simulink model "svpwm"  (R2022b)
settings: Solver=VariableStepAuto  StartTime=0.0  StopTime=10.0  RelTol=1e-3
settings Model: Creator=15403  LastModifiedBy=15403

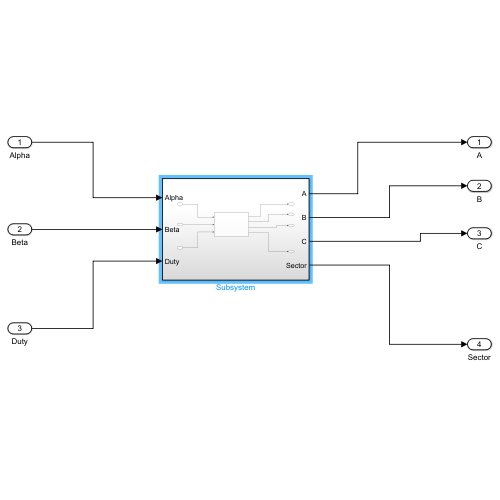
[thumbnail: Simulink's stored preview of the top-level diagram]
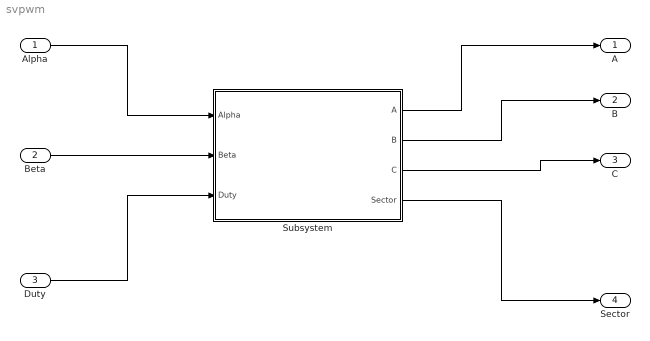
== system svpwm ==
  Alpha : Inport
  Beta : Inport  Port=2
  Duty : Inport  Port=3
  Subsystem : Subsystem
  A : Outport
  B : Outport  Port=2
  C : Outport  Port=3
  Sector : Outport  Port=4
  wires:
  Alpha/1 -> Subsystem/1(Alpha)
  Beta/1 -> Subsystem/2(Beta)
  Duty/1 -> Subsystem/3(Duty)
  Subsystem/1(A) -> A/1
  Subsystem/2(B) -> B/1
  Subsystem/3(C) -> C/1
  Subsystem/4(Sector) -> Sector/1

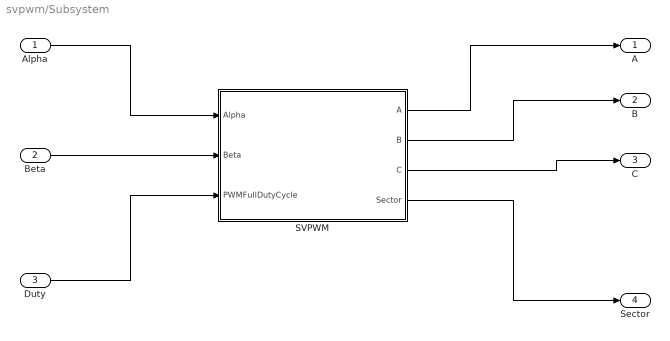
== system svpwm/Subsystem ==
  Alpha : Inport
  Beta : Inport  Port=2
  Duty : Inport  Port=3
  SVPWM : MATLAB Function  TreatAsAtomicUnit=on
  A : Outport
  B : Outport  Port=2
  C : Outport  Port=3
  Sector : Outport  Port=4
  wires:
  SVPWM/1(A) -> A/1
  Duty/1 -> SVPWM/3(PWMFullDutyCycle)
  Alpha/1 -> SVPWM/1(Alpha)
  Beta/1 -> SVPWM/2(Beta)
  SVPWM/3(C) -> C/1
  SVPWM/4(Sector) -> Sector/1
  SVPWM/2(B) -> B/1

== matlab function svpwm/Subsystem/SVPWM ==
  data: Alpha input; A output; B output; C output; Sector output; Beta input; PWMFullDutyCycle input
function [A, B, C, Sector] = fcn(Alpha, Beta, PWMFullDutyCycle)

% 初始化变量
A = 0;
B = 0;
C = 0;                                  
Sector = 0;
ONE_BY_SQRT3 = tand(30);
TWO_BY_SQRT3 = (2.0 * 0.57735026919);

% 扇区判断
if Beta >= 0.0
    if Alpha >= 0.0
        if (ONE_BY_SQRT3 * Beta) > Alpha
                Sector = 2;
        else
            Sector = 1;
        end
    else
        if -ONE_BY_SQRT3 * Beta > Alpha
            Sector = 3;
        else
            Sector = 2;
        end
    end
else
    if Alpha >= 0.0
        if -ONE_BY_SQRT3 * Beta > Alpha
            Sector = 5;
        else
            Sector = 6;
        end

    else
        if ONE_BY_SQRT3 * Beta > Alpha
            Sector = 4;
        else
            Sector = 5;
        end
    end
end


switch Sector
    case 1
        t1 = (Alpha - ONE_BY_SQRT3 * Beta) * PWMFullDutyCycle;
        t2 = (TWO_BY_SQRT3 * Beta) * PWMFullDutyCycle;

        A = (PWMFullDutyCycle + t1 + t2) / 2;
        B = A - t1;
        C = B - t2;
    case 2
		t2 = (Alpha + ONE_BY_SQRT3 * Beta) * PWMFullDutyCycle;
		t3 = (-Alpha + ONE_BY_SQRT3 * Beta) * PWMFullDutyCycle;

		A = (PWMFullDutyCycle + t2 + t3) / 2;
		B = A - t3;
		C = A - t2;
        
    case 3
       t3 = (TWO_BY_SQRT3 * Beta) * PWMFullDutyCycle;
		t4 = (-Alpha - ONE_BY_SQRT3 * Beta) * PWMFullDutyCycle;

		B = (PWMFullDutyCycle + t3 + t4) / 2;
		C = B - t3;
		A = C - t4;

    case 4
		t4 = (-Alpha + ONE_BY_SQRT3 * Beta) * PWMFullDutyCycle;
		t5 = (-TWO_BY_SQRT3 * Beta) * PWMFullDutyCycle;

		C = (PWMFullDutyCycle + t4 + t5) / 2;
		B = C - t5;
		A = B - t4;
    case 5
        t5 = (-Alpha - ONE_BY_SQRT3 * Beta) * PWMFullDutyCycle;
		t6 = (Alpha - ONE_BY_SQRT3 * Beta) * PWMFullDutyCycle;

		C = (PWMFullDutyCycle + t5 + t6) / 2;
		A = C - t5;
		B = A - t6;

    case 6
		t6 = (-TWO_BY_SQRT3 * Beta) * PWMFullDutyCycle;
		t1 = (Alpha + ONE_BY_SQRT3 * Beta) * PWMFullDutyCycle;

		A = (PWMFullDutyCycle + t6 + t1) / 2;
		C = A - t1;
		B = C - t6;
end
